simulink model "Assignment1"  (R2019a)
settings: Solver=FixedStepDiscrete  StartTime=0.0  StopTime=6  FixedStep=1  RelTol=1e-3
libraries: simulink x1
settings Model: Creator=Acer  LastModifiedBy=Acer

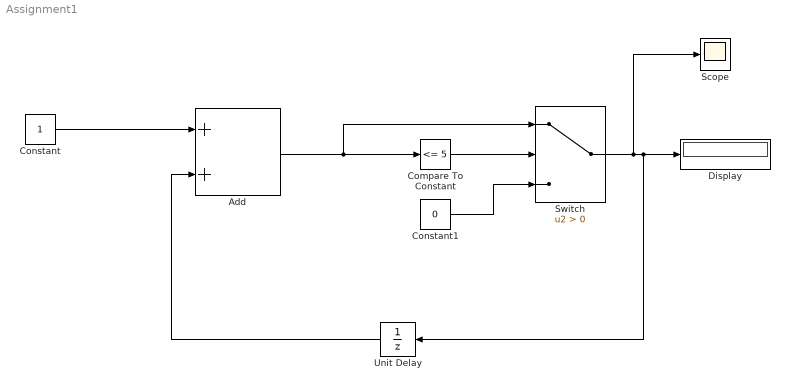
== system Assignment1 ==
  Add : Sum
  Compare To Constant : simulink/Logic and Bit Operations/Compare To Constant  relop=<=  const=5  OutDataTypeStr=boolean
  Constant : Constant
  Constant1 : Constant  Value=0
  Display : Display
  Scope : Scope
  Switch : Switch  Criteria=u2 > Threshold
  Unit Delay : UnitDelay  InitialCondition=-1  SampleTime=-1  HasFrameUpgradeWarning=on
  wires:
  Switch/1 -> Scope/1, Unit Delay/1, Display/1
  Compare To Constant/1 -> Switch/2
  Add/1 -> Switch/1, Compare To Constant/1
  Constant/1 -> Add/1
  Unit Delay/1 -> Add/2
  Constant1/1 -> Switch/3
